simulink library "ac_controller"  (R2023b)
settings: Solver=VariableStepAuto  StartTime=0.0  StopTime=10.0  RelTol=1e-3
undefined symbols (not defined in the file): DiscIntNeverNeededParam, K_p, T_n
settings Model: Creator=mueller.chris-it22  LastModifiedBy=mueller.chris-it22

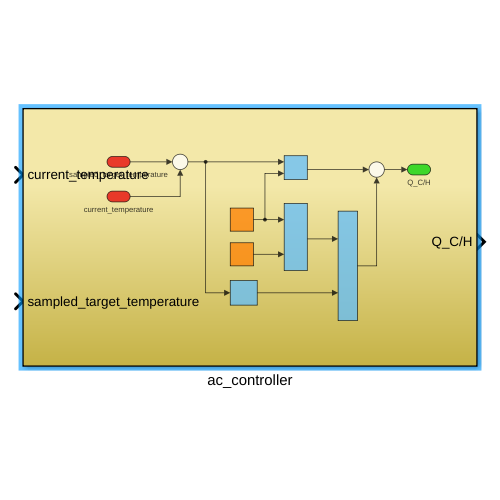
[thumbnail: Simulink's stored preview of the top-level diagram]
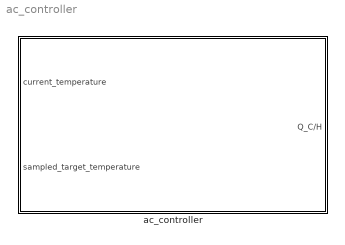
== system ac_controller ==
  ac_controller : Subsystem

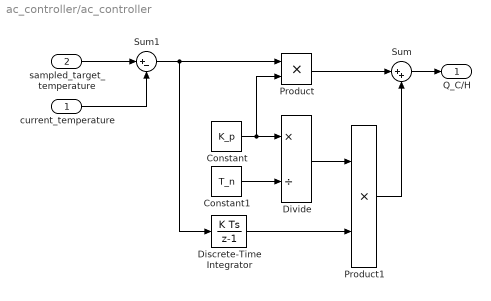
== system ac_controller/ac_controller ==
  current_temperature : Inport  OutDataTypeStr=int16
  sampled_target_temperature : Inport  Port=2  OutDataTypeStr=uint16
  Constant : Constant  Value=K_p  OutDataTypeStr=uint16
  Constant1 : Constant  Value=T_n  OutDataTypeStr=uint16
  Discrete-Time Integrator : DiscreteIntegrator  SampleTime=-1  ICPrevOutput=DiscIntNeverNeededParam  ICPrevScaledInput=DiscIntNeverNeededParam
  Divide : Product  Inputs=*/
  Product : Product
  Product1 : Product
  Sum : Sum  Inputs=|++
  Sum1 : Sum  Inputs=|+-
  Q_C/H : Outport
  wires:
  Discrete-Time Integrator/1 -> Product1/2
  Product/1 -> Sum/1
  Product1/1 -> Sum/2
  Sum1/1 -> Discrete-Time Integrator/1, Product/1
  sampled_target_temperature/1 -> Sum1/1
  current_temperature/1 -> Sum1/2
  Constant/1 -> Product/2, Divide/1
  Constant1/1 -> Divide/2
  Divide/1 -> Product1/1
  Sum/1 -> Q_C/H/1
